simulink model "idmdl"  (R2022a)
settings: Solver=VariableStepAuto  StartTime=0.0  StopTime=10.0  RelTol=1e-3
undefined symbols (not defined in the file): jp, kt, kv, l
libraries: simulink_extras x1
settings Model: Creator=mfussi  LastModifiedBy=mfussi

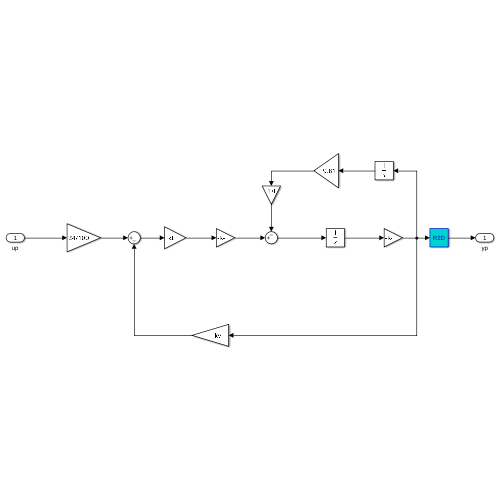
[thumbnail: Simulink's stored preview of the top-level diagram]
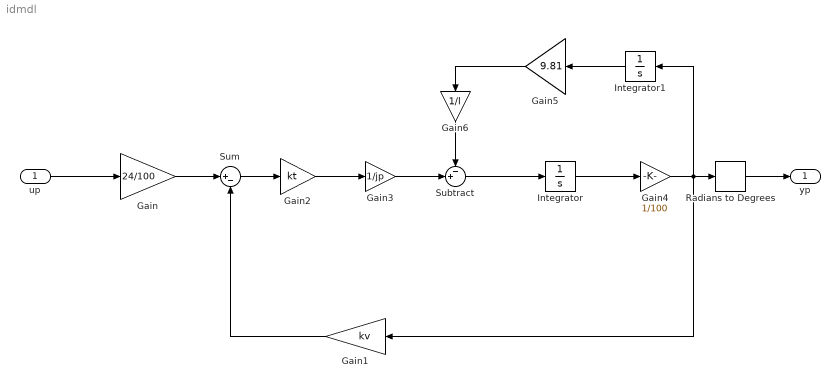
== system idmdl ==
  up : Inport
  Gain : Gain  Gain=24/100
  Gain1 : Gain  Gain=kv
  Gain2 : Gain  Gain=kt
  Gain3 : Gain  Gain=1/jp
  Gain4 : Gain  Gain=1/100
  Gain5 : Gain  Gain=9.81
  Gain6 : Gain  Gain=1/l
  Integrator : Integrator
  Integrator1 : Integrator
  Radians to Degrees : simulink_extras/Transformations/Radians to Degrees
  Subtract : Sum  Inputs=-+|
  Sum : Sum  Inputs=|+-
  yp : Outport
  wires:
  up/1 -> Gain/1
  Gain/1 -> Sum/1
  Gain1/1 -> Sum/2
  Sum/1 -> Gain2/1
  Integrator/1 -> Gain4/1
  Gain3/1 -> Subtract/2
  Radians to Degrees/1 -> yp/1
  Gain4/1 -> Gain1/1, Integrator1/1, Radians to Degrees/1
  Gain2/1 -> Gain3/1
  Subtract/1 -> Integrator/1
  Integrator1/1 -> Gain5/1
  Gain5/1 -> Gain6/1
  Gain6/1 -> Subtract/1
